simulink subsystem "delay"  (R2024a)
settings: Solver=VariableStepAuto  StartTime=0.0  StopTime=10.0  RelTol=1e-3
model mask{delay_type="none", delay_value=delay_value, bus=bus, BusTemplate=BusTemplate, BusInitialValue=BusInitialValue}
  mask prompts: delay_type "Delay Type"; delay_value "Delay Value"; BusTemplate "Bus Template"; BusInitialValue "Bus Initial Value"
undefined symbols (not defined in the file): populateVectorFromNumericStructure
settings Model: Creator=Friedrich Tuttas  LastModifiedBy=Friedrich Tuttas

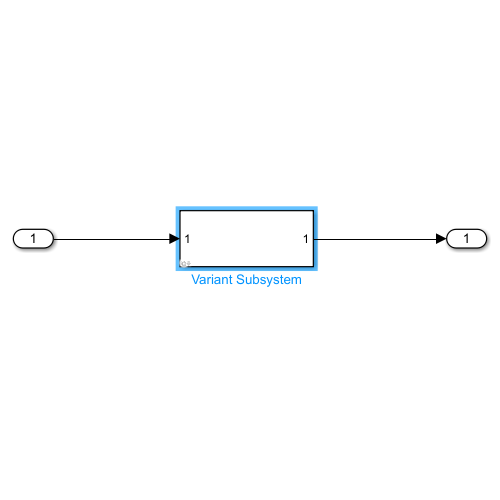
[thumbnail: Simulink's stored preview of the top-level diagram]
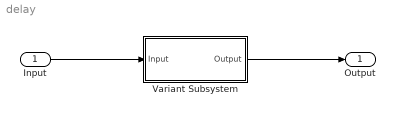
== system delay ==
  Input : Inport
  Variant Subsystem : Subsystem  Variant=on  mask{delay_value=delay_value, bus=bus, BusTemplate=BusTemplate, BusInitialValue=BusInitialValue}
      mask prompts: delay_value "Delay Value"; BusTemplate "Bus Template"; BusInitialValue "Bus Initial Value"
      mask TypeOptions delay_value: Continuous/delay_value | Discrete/delay_value
      mask TypeOptions bus: Continuous/bus
      mask TypeOptions BusTemplate: Continuous/BusTemplate
      mask TypeOptions BusInitialValue: Continuous/BusInitialValue | Discrete/BusInitialValue
  Output : Outport
  wires:
  Variant Subsystem/1(Output) -> Output/1
  Input/1 -> Variant Subsystem/1(Input)

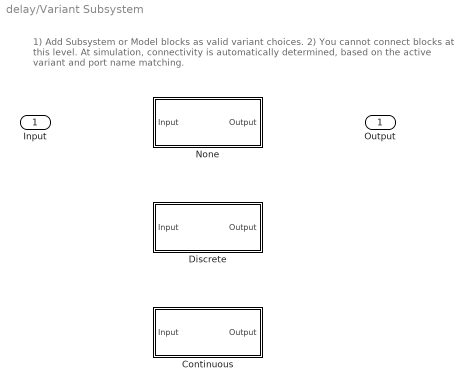
== system delay/Variant Subsystem ==
  note: 1) Add Subsystem or Model blocks as valid variant choices.
      | 2) You cannot connect blocks at this level. At simulation, connectivity is automatically
      | determined, based on the active variant and port name matching.
  Input : Inport
  Continuous : Subsystem  VariantControl="delay_type == \"continuous\""  mask{delay_value=delay_value, bus=bus, BusTemplate=BusTemplate, BusInitialValue=BusInitialValue}
      mask prompts: delay_value "Delay Value"; BusTemplate "Bus Template"; BusInitialValue "Bus Initial Value"
      mask TypeOptions bus: Subsystem Reference/bus
      mask TypeOptions BusTemplate: Subsystem Reference/BusTemplate
  Discrete : Subsystem  VariantControl="delay_type == \"discrete\""  mask{delay_value=delay_value, BusInitialValue=BusInitialValue}
      mask prompts: delay_value "Delay Value"; BusInitialValue "Bus Initial Value"
  None : Subsystem  VariantControl="delay_type == \"none\""
  Output : Outport

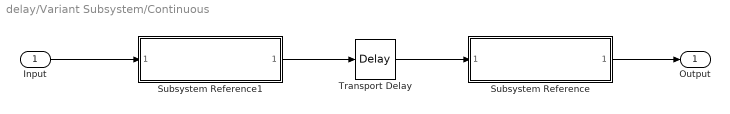
== system delay/Variant Subsystem/Continuous ==
  Input : Inport
  Subsystem Reference : Subsystem  ReferencedSubsystem=bus_from_vector  bus=bus  BusTemplate=BusTemplate
  Subsystem Reference1 : Subsystem  ReferencedSubsystem=vector_from_bus
  Transport Delay : TransportDelay  DelayTime=delay_value  InitialOutput=populateVectorFromNumericStructure(BusInitialValue)
  Output : Outport
  wires:
  Transport Delay/1 -> Subsystem Reference/1
  Input/1 -> Subsystem Reference1/1
  Subsystem Reference1/1 -> Transport Delay/1
  Subsystem Reference/1 -> Output/1

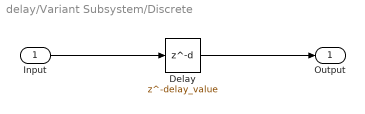
== system delay/Variant Subsystem/Discrete ==
  Input : Inport
  Delay : Delay  DelayLength=delay_value  InitialCondition=BusInitialValue
  Output : Outport
  wires:
  Input/1 -> Delay/1
  Delay/1 -> Output/1

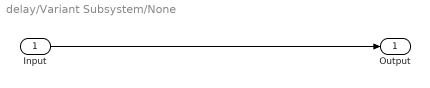
== system delay/Variant Subsystem/None ==
  Input : Inport
  Output : Outport
  wires:
  Input/1 -> Output/1
